simulink model "glucose_insulin_normal"  (R2018a)
settings: Solver=VariableStepAuto  StartTime=0.0  StopTime=10  RelTol=1e-3
libraries: simulink x2
settings Model: Creator=dinet  LastModifiedBy=HP
settings DebuggingCC: LibraryContextMissingDiagnostic=warning
settings SFSimCC: SimUseLocalCustomCode=on
settings RTWCC: RTWUseLocalCustomCode=on

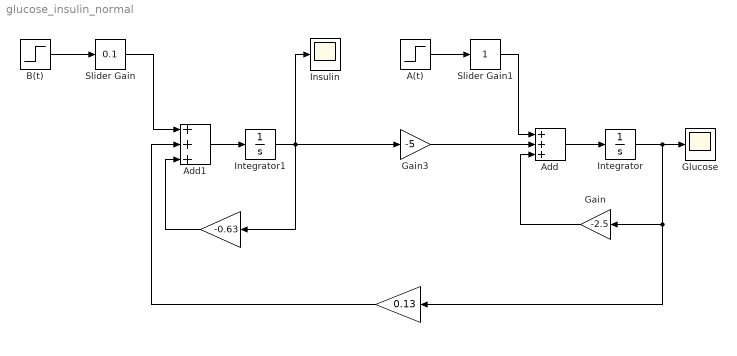
== system glucose_insulin_normal ==
  " " : Gain  Gain=-0.63
  " " : Gain  Gain=0.13
  A(t) : Step  SampleTime=0
  Add : Sum  Inputs=+++
  Add1 : Sum  Inputs=+++
  B(t) : Step  Time=0  SampleTime=0
  Gain : Gain  Gain=-2.5
  Gain3 : Gain  Gain=-5
  Glucose : Scope
  Insulin : Scope
  Integrator : Integrator
  Integrator1 : Integrator
  Slider Gain : simulink/Math Operations/Slider Gain  gain=0.1  low=0  high=2
  Slider Gain1 : simulink/Math Operations/Slider Gain  gain=1  low=0  high=2
  wires:
  B(t)/1 -> Slider Gain/1
  Slider Gain/1 -> Add1/1
  Add1/1 -> Integrator1/1
  Integrator1/1 -> Gain3/1, Insulin/1, " "/1
  Gain3/1 -> Add/2
  A(t)/1 -> Slider Gain1/1
  Slider Gain1/1 -> Add/1
  Gain/1 -> Add/3
  Add/1 -> Integrator/1
  Integrator/1 -> " "/1, Gain/1, Glucose/1
  " "/1 -> Add1/3
  " "/1 -> Add1/2
